simulink library "hapsrav_library"  (R2017a)
settings: Solver=VariableStepAuto  StartTime=0.0  StopTime=10.0  RelTol=1e-3
values from neighbouring files (symbols this model uses):
  absorb_h = 0:100:40000    [EnergySim.m]
  Adisk = pi * v.R_prop^2    [EnergySim.m]
  alpha_h = absorb_h    [EnergySim.m]
  aoa_data = zeros(n_cl, n)    [EnergySim.m]
  cl_bp = linspace(min_cl, max_cl,n_cl)    [EnergySim.m]
  D = [1       -.0065      288.15          0                   101325 ... (first row only)    [EnergySim.m]    (also in msn_params.m = sqrt((from_x - to_x)^2 + (from_y - to_y)^2); solar_vector.m = time.day + ut_time)
  d2r = pi / 180    (= 0.0174532925199)    [EnergySim.m]    (also in example1.m; example2.m; example3.m; example4.m)
  d_init = sqrt(dx*dx + dy*dy)    [EnergySim.m]    (also in msn_init.m)
  dchi0 = atan2(sin(dchi0), cos(dchi0))    [EnergySim.m]    (also in msn_init.m)
  dT = 0.5    [EnergySim.m]
  dT_fixed = 0.5    [EnergySim.m]
  dT_trig = 30    [EnergySim.m]
  earth_rho = 6378137.0    (= 6378137)    [EnergySim.m]
  fp = solarFP(p.orbit_rho, p.min_axis, p.orbit_dir, ic.x_ctr, ic.y_ctr, sun_az_0)    [EnergySim.m]    (also in load_fp.m = gid_tc(msn_idx).fp; solarFP.m = [1	6	2	nul eul 0	0	0	0	1	0)
  fp_coords = [x_entry y_entry]    [msn_params.m]
  fp_courses = [chi_adj nxt_chi dchi]    [msn_params.m]
  g = 9.80665    [EnergySim.m]
  Gsolar = 1367    [EnergySim.m]
  k = k+1    (= 5)    [EnergySim.m]
  K = D(:,2)    [EnergySim.m]
  lat_init = ic.lat_init_deg * obj.d2r    [EnergySim.m]
  M = time.month    [solar_vector.m]
  max_cl = max(cl_data(:))    [EnergySim.m]
  min_cl = min(cl_data(:))    [EnergySim.m]
  ND2 = load(fullfile(pwd,'nd2_data.mat'))    [EnergySim.m]    (also in nd2_data.mat = [0.0999999999999 0.200000000001 0.3 0.4 0.499999999998 0.700)
  next_init = fp(init_wp, 3)    [EnergySim.m]    (also in msn_init.m)
  pE_init = ic.pE_init    [EnergySim.m]
  pN_init = ic.pN_init    [EnergySim.m]
  r2d = 180 / pi    (= 57.2957795131)    [EnergySim.m]    (also in example1.m; example2.m; example3.m; example4.m)
  rho_SL = 1.225    [EnergySim.m]
  S = 110.4    [EnergySim.m]
  thr_lo_lim = 0.0    (= 0)    [EnergySim.m]
  time_init = struct('year', time.year, 'month', time.month,                  'day', time.day, 'hour', time.hour, 'min', time.min,                  'UTC', time.UTC)    [EnergySim.m]
  to_init = fp(init_wp, 1)    [EnergySim.m]    (also in msn_init.m)
  vgnd_init = sqrt(Vg)    [EnergySim.m]
  vtas_init = veas_init * sqrt(rho_sl/rho_alt)    [EnergySim.m]
  w_alt = 2.0 * w_alt    [EnergySim.m]
  w_xtrack = 2.0 * w_xtrack    [EnergySim.m]
undefined symbols (not defined in the file or in its folder): alpha, alpha_bp, alpha_circ, alt0_rate_init, alt_bp, alt_cmd_mode, alt_init, alt_lim_h, alt_lim_l, alt_rt_lim_periodic, cd_data, charge_eff, chi0_rate_init, chi_cmd_mode, chi_inf, chi_init, cl_data, discharge_eff, DiscIntNeverNeededParam, E_batt_max, E_init, Earth, enableFuzzyLogic, entry_init, epsln, epsln_circ, exit_init, f8_azimuth_offset, fig_eight_time, fp0, fp_coords0, fp_courses0, gamma_lim, hold_time, k_c, K_circ, lat_init_deg, lon_init_deg, max_alpha_bp, max_alt_bp, min_alpha_bp, min_alt_bp, min_axis, motor_eff, mppt_eff, num_motors, orb_dir_init, orb_len_init, orbit_dir, orbit_rho, P_acc, panel_eff, panel_vecs, phi_0, phi_lim, phi_lim_alt, phi_lim_alt_max, phi_lim_alt_min, phi_rt_lim, prop_eff_scale ... (+39)
libraries: simulink x59, hapsrav_library x9, fuzblock x3, atmospheric_library x1, aerolibtransform2 x1
(part 5 of 6)

== system hapsrav_library/hapsrav_main/Kinematic 6DOF/Selectable Modes/Waypoint_Navigation/Altitude/alt_rate ==
  max_clmb_rt : Inport
  max_desc_rt : Inport  Port=2
  d2alt : Inport  Port=3
  altRt0 : Inport  Port=4
  idleDesc : Inport  Port=5
  Constant : Constant  Value=dT
  Freezable Limited Integration1 : hapsrav_library/Freezable Limited Integration
  Mux : Mux  Inputs=2
  Scope : Scope
  d1alt : Outport
  wires:
  [dn_lim] -> Freezable Limited Integration1/6
  max_clmb_rt/1 -> [up_lim]
  max_desc_rt/1 -> [dn_lim]
  idleDesc/1 -> Freezable Limited Integration1/4
  altRt0/1 -> Freezable Limited Integration1/3
  [up_lim] -> Freezable Limited Integration1/5
  Constant/1 -> Freezable Limited Integration1/2
  d2alt/1 -> Freezable Limited Integration1/1
  Freezable Limited Integration1/1 -> Mux/1, d1alt/1
  Mux/1 -> Scope/1
  [dn_lim] -> Mux/2

== system hapsrav_library/hapsrav_main/Kinematic 6DOF/Selectable Modes/Waypoint_Navigation/Course/Circular Integration ==
  u : Inport
  x0 : Inport  Port=2
  Discrete-Time Integrator : DiscreteIntegrator  Commented=on  IntegratorMethod=Integration: Trapezoidal  InitialConditionSource=external  InitialConditionSetting=State (most efficient)  SampleTime=-1  ICPrevOutput=DiscIntNeverNeededParam  ICPrevScaledInput=DiscIntNeverNeededParam
  Integrator : Integrator  InitialConditionSource=external  WrapState=on
  Trigonometric Function : Trigonometry  Commented=on  Operator=sincos
  Trigonometric Function1 : Trigonometry  Commented=on  Operator=atan2
  y : Outport
  wires:
  Integrator/1 -> y/1
  u/1 -> Integrator/1
  x0/1 -> Integrator/2
  Discrete-Time Integrator/1 -> Trigonometric Function/1
  Trigonometric Function/2 -> Trigonometric Function1/2
  Trigonometric Function/1 -> Trigonometric Function1/1

== system hapsrav_library/hapsrav_main/Kinematic 6DOF/Selectable Modes/Waypoint_Navigation/Course/Rate Limits ==
  Vg : Inport
  alt : Inport  Port=2
  d2chi : Inport  Port=3
  d1Vg : Inport  Port=4
  Divide : Product  Inputs=*/
  Divide1 : Product  Inputs=*/
  Divide2 : Product  Inputs=**
  Divide3 : Product  Inputs=**
  Gain : Gain  Gain=g
  Gain1 : Gain  Gain=g
  Gain2 : Gain  Gain=-1
  Math Function : Math  Operator=reciprocal  SaturateOnIntegerOverflow=on
  Math Function1 : Math  Operator=square  SaturateOnIntegerOverflow=on
  Math Function2 : Math  Operator=square  SaturateOnIntegerOverflow=on
  Saturation : Saturate  UpperLimit=phi_lim_alt_max  LowerLimit=phi_lim_alt_min
  Saturation Dynamic : simulink/Discontinuities/Saturation Dynamic  OutMin=[]  OutMax=[]  OutDataTypeStr=Inherit: Same as second input  OutDataType=fixdt(1, 16)  OutScaling=2^-10  DoSatur=off
  Sum : Sum  Inputs=|-+
  Trigonometric Function : Trigonometry  Operator=tan
  Trigonometric Function1 : Trigonometry  Operator=cos
  phi_lim LUT : Lookup_n-D  NumberOfTableDimensions=1  BreakpointsForDimension1=phi_lim_alt  Table=phi_lim  ExtrapMethod=Clip  DiagnosticForOutOfRangeInput=Error  RemoveProtectionInput=on  UseLastTableValue=on  InternalRulePriority=Speed  RndMeth=Simplest  InputSameDT=on
  phi_rt_lim LUT : Lookup_n-D  NumberOfTableDimensions=1  BreakpointsForDimension1=phi_lim_alt  Table=phi_rt_lim  ExtrapMethod=Clip  DiagnosticForOutOfRangeInput=Error  RemoveProtectionInput=on  UseLastTableValue=on  InternalRulePriority=Speed  RndMeth=Simplest  InputSameDT=on
  phi_lim : Outport
  d2chi_lim : Outport  Port=2
  wires:
  d2chi/1 -> Saturation Dynamic/2
  Saturation Dynamic/1 -> d2chi_lim/1
  [phi_lim] -> Trigonometric Function/1
  Trigonometric Function/1 -> Gain/1
  Gain/1 -> Divide/1
  Math Function2/1 -> Divide/2
  Vg/1 -> [Vg]
  [Vg] -> Math Function2/1
  Trigonometric Function1/1 -> Math Function/1
  Math Function/1 -> Math Function1/1
  Math Function1/1 -> Gain1/1
  Gain1/1 -> Divide1/1
  [Vg] -> Divide1/2
  Divide1/1 -> Divide2/2
  Divide2/1 -> Sum/2
  Sum/1 -> [up_lim]
  [up_lim] -> Saturation Dynamic/1
  [up_lim] -> Gain2/1
  Gain2/1 -> Saturation Dynamic/3
  Divide/1 -> Divide3/2
  Divide3/1 -> Sum/1
  alt/1 -> Saturation/1
  [alt] -> phi_lim LUT/1
  phi_lim LUT/1 -> [phi_lim]
  [phi_lim] -> Trigonometric Function1/1
  [alt] -> phi_rt_lim LUT/1
  phi_rt_lim LUT/1 -> [phi_rt_lim]
  [phi_rt_lim] -> Divide2/1
  [phi_lim] -> phi_lim/1
  Saturation/1 -> [alt]
  d1Vg/1 -> Divide3/1

== system hapsrav_library/hapsrav_main/Kinematic 6DOF/Selectable Modes/Waypoint_Navigation/Course/Wrap +//- pi ==
  ang : Inport
  Trigonometric Function : Trigonometry  Operator=sincos
  Trigonometric Function1 : Trigonometry  Operator=atan2
  ang_pi : Outport
  wires:
  ang/1 -> Trigonometric Function/1
  Trigonometric Function/1 -> Trigonometric Function1/1
  Trigonometric Function/2 -> Trigonometric Function1/2
  Trigonometric Function1/1 -> ang_pi/1

== system hapsrav_library/hapsrav_main/Kinematic 6DOF/Selectable Modes/Waypoint_Navigation/Course/chi_dot ==
  Vg : Inport
  phi_lim : Inport  Port=2
  d2chi : Inport  Port=3
  Constant : Constant  Value=dT
  Constant1 : Constant  Value=g
  Constant2 : Constant  Value=chi0_rate_init
  Delay1 : Delay  DelayLength=1  InitialConditionSource=Input port
      settings: InputPortMap=u0,p4
  Divide : Product  Inputs=*/
  Divide1 : Product  Inputs=**
  Divide2 : Product  Inputs=**
  Gain : Gain  Gain=1/g
  Limited Integration : MATLAB Function  TreatAsAtomicUnit=on
  Trigonometric Function : Trigonometry  Operator=tan
  Trigonometric Function1 : Trigonometry  Operator=atan
  phi : Outport
  d1chi : Outport  Port=2
  wires:
  Constant/1 -> Limited Integration/2(T)
  Delay1/1 -> Limited Integration/4(x0)
  Limited Integration/2(x1) -> Delay1/1
  Limited Integration/1(y0) -> d1chi/1, Divide2/1
  d2chi/1 -> Limited Integration/1(u)
  Constant1/1 -> Divide/1
  Divide/1 -> Divide1/1
  phi_lim/1 -> Trigonometric Function/1
  Trigonometric Function/1 -> Divide1/2
  Divide1/1 -> [rate_lim]
  [rate_lim] -> Limited Integration/3(lim)
  Vg/1 -> [Vg]
  [Vg] -> Divide/2
  [Vg] -> Divide2/2
  Divide2/1 -> Gain/1
  Gain/1 -> Trigonometric Function1/1
  Trigonometric Function1/1 -> phi/1
  Constant2/1 -> Delay1/2

== system hapsrav_library/hapsrav_main/Kinematic 6DOF/Selectable Modes/Waypoint_Navigation/Lat Cmd Filter/Filtered Command ==
  chi cmd : Inport
  chi_init : Inport  Port=2
  Enable : EnablePort
  1/tau : Gain  Gain=0.1
  Delay1 : Delay  DelayLength=1  InitialConditionSource=Input port
      settings: InputPortMap=u0,p4
  Discrete-Time Integrator : DiscreteIntegrator  IntegratorMethod=Integration: Trapezoidal  InitialConditionSource=external  InitialConditionSetting=State (most efficient)  SampleTime=-1  ICPrevOutput=DiscIntNeverNeededParam  ICPrevScaledInput=DiscIntNeverNeededParam
  Sum : Sum  Inputs=|+-
  filt chi cmd : Outport
  wires:
  chi cmd/1 -> Sum/1
  [chi_init] -> Delay1/2
  1/tau/1 -> Discrete-Time Integrator/1
  chi_init/1 -> [chi_init]
  Sum/1 -> 1/tau/1
  Discrete-Time Integrator/1 -> filt chi cmd/1, Delay1/1
  [chi_init] -> Discrete-Time Integrator/2
  Delay1/1 -> Sum/2

== system hapsrav_library/hapsrav_main/Kinematic 6DOF/Selectable Modes/Waypoint_Navigation/Lat Cmd Filter/Unfiltered Command ==
  cmd : Inport
  Enable : EnablePort
  cmdFilt : Outport
  wires:
  cmd/1 -> cmdFilt/1

== system hapsrav_library/Cmd - Parametric/Chi Cmd/Flight Plan/Mission Command/Entry Mode/Desired Course/Desired Course ==
  xtrack : Inport
  Gain3 : Gain  Gain=k
  Gain5 : Gain  Gain=2/pi
  Gain6 : Gain  Gain=chi_inf
  Gain7 : Gain  Gain=-1
  Trigonometric Function1 : Trigonometry  Operator=atan
  chi_d : Outport
  wires:
  Gain7/1 -> chi_d/1
  Gain6/1 -> Gain7/1
  Trigonometric Function1/1 -> Gain5/1
  Gain3/1 -> Trigonometric Function1/1
  Gain5/1 -> Gain6/1
  xtrack/1 -> Gain3/1

== system hapsrav_library/Cmd - Parametric/Chi Cmd/Flight Plan/Mission Command/Entry Mode/xtrack Error/Distance ==
  to_x : Inport
  from_x : Inport  Port=2
  to_y : Inport  Port=3
  from_y : Inport  Port=4
  Product of Elements : Product
  Product of Elements1 : Product
  Sqrt : Sqrt  SaturateOnIntegerOverflow=on
  Sum : Sum  Inputs=|+-
  Sum1 : Sum  Inputs=|+-
  Sum2 : Sum  Inputs=|++
  Dist : Outport
  wires:
  Sum1/1 -> [dy]
  to_x/1 -> Sum/1
  Sum/1 -> [dx]
  from_y/1 -> Sum1/2
  to_y/1 -> Sum1/1
  Sqrt/1 -> Dist/1
  Sum2/1 -> Sqrt/1
  [dx] -> Product of Elements/1, Product of Elements/2
  Product of Elements1/1 -> Sum2/2
  Product of Elements/1 -> Sum2/1
  [dy] -> Product of Elements1/1, Product of Elements1/2
  from_x/1 -> Sum/2

== system hapsrav_library/Cmd - Parametric/Chi Cmd/Flight Plan/Mission Command/Not Entry Mode/Circular Pattern Holding/Sweep Angle ==
  av_y : Inport
  y_ctr : Inport  Port=2
  av_x : Inport  Port=3
  x_ctr : Inport  Port=4
  Abs : Abs
  Abs1 : Abs
  Abs2 : Abs
  Counter Free-Running : simulink/Sources/Counter Free-Running  NumBits=32  tsamp=-1
  Delay : Delay  DelayLength=1  InitialConditionSource=Input port
      settings: InputPortMap=u0,p4
  Memory : Memory
  Memory3 : Memory
  Sum1 : Sum  Inputs=|+-
  Sum2 : Sum  Inputs=|+-
  Sum3 : Sum  Inputs=|+-
  Sum4 : Sum  Inputs=|++
  Switch : Switch  Criteria=u2 ~= 0
  Trigonometric Function1 : Trigonometry  Operator=atan2
  swept_angle : Outport
  wires:
  Memory/1 -> Sum4/2
  Abs/1 -> Delay/2
  Sum1/1 -> Abs2/1
  [rel_hdg] -> Switch/3
  Sum3/1 -> Trigonometric Function1/1
  Abs2/1 -> Sum4/1
  Trigonometric Function1/1 -> [rel_hdg]
  Sum2/1 -> Trigonometric Function1/2
  [rel_hdg] -> Abs1/1
  Sum4/1 -> Memory/1, swept_angle/1
  Delay/1 -> Sum1/2
  [rel_hdg_0] -> Abs/1
  Counter Free-Running/1 -> Switch/2
  y_ctr/1 -> Sum3/2
  av_x/1 -> Sum2/1
  x_ctr/1 -> Sum2/2
  av_y/1 -> Sum3/1
  Abs1/1 -> Sum1/1, Delay/1
  Memory3/1 -> Switch/1
  Switch/1 -> Memory3/1, [rel_hdg_0]

== system hapsrav_library/Cmd - Parametric/Chi Cmd/Flight Plan/Mission Command/Not Entry Mode/Linear Following/Path Following ==
  leg_coords : Inport
  leg_crs : Inport  Port=2
  av_state : Inport  Port=3
  Bus Selector1 : BusSelector  OutputSignals=av_posn,av_course,av_gndspeed
  Constant1 : Constant  Value=alpha
  Constant2 : Constant  Value=epsln
  Constant3 : Constant  Value=k
  Constant4 : Constant  Value=K
  Constant5 : Constant  Value=chi_inf
  Course : Subsystem  TreatAsAtomicUnit=on
  Desired Course : Subsystem  TreatAsAtomicUnit=on
  Logical Operator : Logic  Operator=NOT  AllPortsSameDT=off  OutDataTypeStr=boolean
  MATLAB Function : MATLAB Function  TreatAsAtomicUnit=on
  Merge1 : Merge
  xtrack Error : Subsystem  TreatAsAtomicUnit=on
  chi_cmd : Outport
  chi_d : Outport  Port=2
  xtrack : Outport  Port=3
  wires:
  [chi_d] -> chi_d/1
  Merge1/1 -> [chi_d]
  [chi_d_0] -> Merge1/2
  [chi_d_1] -> Merge1/1
  Course/1(chi_d) -> [chi_d_0]
  [av_posn] -> Course/2(av_posn)
  [leg_coords] -> Course/1(leg_coords)
  [leg_coords] -> xtrack Error/1(leg_coords)
  leg_coords/1 -> [leg_coords]
  [collocated] -> Course/Enable
  [collocated] -> Logical Operator/1
  Logical Operator/1 -> Desired Course/Enable
  xtrack Error/2(collacated) -> [collocated]
  leg_crs/1 -> Desired Course/1(leg_crs)
  [xtrack] -> xtrack/1
  [xtrack] -> Desired Course/2(xtrack)
  Desired Course/1(chi_d) -> [chi_d_1]
  xtrack Error/1(xtrk) -> [xtrack]
  [av_posn] -> xtrack Error/2(av_posn)
  Bus Selector1/1 -> [av_posn]  "<av_posn>"
  [Vg] -> MATLAB Function/4(Vg)
  [chi] -> MATLAB Function/1(chi)
  Bus Selector1/3 -> [Vg]  "<av_gndspeed>"
  av_state/1 -> Bus Selector1/1
  Bus Selector1/2 -> [chi]  "<av_course>"
  Constant5/1 -> MATLAB Function/5(chi_inf)
  Constant3/1 -> MATLAB Function/8(k)
  [chi_d] -> MATLAB Function/2(chi_d)
  [xtrack] -> MATLAB Function/3(xtrack)
  Constant2/1 -> MATLAB Function/7(e)
  Constant1/1 -> MATLAB Function/6(alpha)
  Constant4/1 -> MATLAB Function/9(K)
  MATLAB Function/1(chi_cmd) -> chi_cmd/1

== system hapsrav_library/Cmd - Parametric/Chi Cmd/Flight Plan/Mission Director/Nav Leg/Flight Plan/Realtime FP ==
  sol_az : Inport  PortDimensions=1
  Enable : EnablePort
  Constant4 : Constant  Value=orbit_rho  VectorParams1D=off  OutDataTypeStr=double
  Constant5 : Constant  Value=min_axis  VectorParams1D=off  OutDataTypeStr=double
  Constant6 : Constant  Value=orbit_dir  VectorParams1D=off  OutDataTypeStr=boolean
  Constant7 : Constant  Value=x_ctr  VectorParams1D=off  OutDataTypeStr=double
  Constant8 : Constant  Value=y_ctr  VectorParams1D=off  OutDataTypeStr=double
  MATLAB Function : MATLAB Function  TreatAsAtomicUnit=on
  Trigonometric Function : Trigonometry  Operator=sincos  OutputSignalType=real
  Trigonometric Function1 : Trigonometry  Operator=atan2  OutputSignalType=real
  fp : Outport  PortDimensions=[6,11]  InitialOutput=fp0
  fp_courses : Outport  Port=2  PortDimensions=[6,3]  InitialOutput=fp_courses0
  fp_coords : Outport  Port=3  PortDimensions=[6,2]  InitialOutput=fp_coords0
  wires:
  sol_az/1 -> Trigonometric Function/1
  MATLAB Function/3(fp_coords) -> fp_coords/1
  MATLAB Function/2(fp_courses) -> fp_courses/1
  Trigonometric Function1/1 -> MATLAB Function/6(az)
  Trigonometric Function/2 -> Trigonometric Function1/2
  Trigonometric Function/1 -> Trigonometric Function1/1
  Constant8/1 -> MATLAB Function/5(y_ctr)
  Constant5/1 -> MATLAB Function/2(min_axis)
  Constant7/1 -> MATLAB Function/4(x_ctr)
  Constant4/1 -> MATLAB Function/1(maj_axis)
  Constant6/1 -> MATLAB Function/3(orbit_dir)
  MATLAB Function/1(fp) -> fp/1

== system hapsrav_library/Cmd - Parametric/Chi Cmd/Flight Plan/Mission Director/Nav Leg/WP Coords/Course ==
  to wp : Inport
  fp_courses : Inport  Port=2
  Assignment1 : Assignment  DiagnosticForDimensions=Warning  IndexOptions=Index vector (port)  Indices=1  OutputSizes=1
  Constant3 : Constant  Value=sel_vec
  Constant4 : Constant
  Demux1 : Demux  Outputs=3
  Gain1 : Gain  Commented=on  Gain=fp_courses  Multiplication=Matrix(u*K)
  Product : Product  Multiplication=Matrix(*)
  Reshape : Reshape  OutputDimensionality=Row vector (2-D)
  Terminator : Terminator
  Terminator1 : Terminator
  next_leg_crs : Outport
  wires:
  fp_courses/1 -> Product/2
  Product/1 -> Demux1/1
  Reshape/1 -> Product/1
  Assignment1/1 -> Reshape/1
  Demux1/3 -> Terminator1/1  "delta_crs"
  to wp/1 -> Assignment1/3
  Constant3/1 -> Assignment1/1
  Constant4/1 -> Assignment1/2
  Demux1/2 -> next_leg_crs/1
  Demux1/1 -> Terminator/1  "leg_crs"

== system hapsrav_library/Cmd - Parametric/Chi Cmd/Flight Plan/Mission Director/Nav Leg/WP Coords/From WP ==
  to wp : Inport
  fp_coords : Inport  Port=2
  Assignment1 : Assignment  DiagnosticForDimensions=Warning  IndexOptions=Index vector (port)  Indices=1  OutputSizes=1
  Constant3 : Constant  Value=sel_vec
  Constant4 : Constant
  Demux1 : Demux  Outputs=2
  Gain1 : Gain  Commented=on  Gain=fp_coords  Multiplication=Matrix(u*K)
  Product : Product  Multiplication=Matrix(*)
  Reshape : Reshape  OutputDimensionality=Row vector (2-D)
  out_x : Outport
  out_y : Outport  Port=2
  wires:
  fp_coords/1 -> Product/2
  Product/1 -> Demux1/1
  Reshape/1 -> Product/1
  Assignment1/1 -> Reshape/1
  to wp/1 -> Assignment1/3
  Constant3/1 -> Assignment1/1
  Constant4/1 -> Assignment1/2
  Demux1/2 -> out_y/1
  Demux1/1 -> out_x/1

== system hapsrav_library/Cmd - Parametric/Chi Cmd/Flight Plan/Mission Director/Nav Leg/WP Coords/To WP ==
  to wp : Inport
  fp_coords : Inport  Port=2
  Assignment1 : Assignment  DiagnosticForDimensions=Warning  IndexOptions=Index vector (port)  Indices=1  OutputSizes=1
  Constant3 : Constant  Value=sel_vec
  Constant4 : Constant
  Demux1 : Demux  Outputs=2
  Gain1 : Gain  Commented=on  Gain=fp_coords  Multiplication=Matrix(u*K)
  Product : Product  Multiplication=Matrix(*)
  Reshape : Reshape  OutputDimensionality=Row vector (2-D)
  out_x : Outport
  out_y : Outport  Port=2
  wires:
  Product/1 -> Demux1/1
  fp_coords/1 -> Product/2
  Reshape/1 -> Product/1
  Assignment1/1 -> Reshape/1
  Demux1/1 -> out_x/1
  Demux1/2 -> out_y/1
  Constant4/1 -> Assignment1/2
  Constant3/1 -> Assignment1/1
  to wp/1 -> Assignment1/3

== system hapsrav_library/Cmd - Parametric/Chi Cmd/Flight Plan/Mission Command/Not Entry Mode/Linear Following/Path Following/Course ==
  leg_coords : Inport
  av_posn : Inport  Port=2
  Enable : EnablePort
  Demux1 : Demux
  Demux2 : Demux
  Sum : Sum  Inputs=|+-
  Sum1 : Sum  Inputs=|+-
  Terminator{,1..3} (4 alike) : Terminator
  Trigonometric Function : Trigonometry  Operator=atan2
  chi_d : Outport
  wires:
  Trigonometric Function/1 -> chi_d/1
  Sum1/1 -> Trigonometric Function/2
  Sum/1 -> Trigonometric Function/1
  [av_x] -> Sum1/2
  [x1] -> Sum1/1
  [av_y] -> Sum/2
  [y1] -> Sum/1
  Demux1/4 -> Terminator1/1
  Demux1/3 -> Terminator/1
  av_posn/1 -> Demux1/1
  Demux1/2 -> [av_y]
  Demux1/1 -> [av_x]
  leg_coords/1 -> Demux2/1
  Demux2/4 -> Terminator3/1
  Demux2/3 -> Terminator2/1
  Demux2/2 -> [y1]
  Demux2/1 -> [x1]

== system hapsrav_library/Cmd - Parametric/Chi Cmd/Flight Plan/Mission Command/Not Entry Mode/Linear Following/Path Following/Desired Course ==
  leg_crs : Inport
  xtrack : Inport  Port=2
  Enable : EnablePort
  Desired Course : Subsystem
  Sum : Sum  Inputs=|++
  chi_d : Outport
  wires:
  leg_crs/1 -> Sum/1
  xtrack/1 -> Desired Course/1(xtrack)
  Sum/1 -> chi_d/1
  Desired Course/1(chi_d) -> Sum/2

== system hapsrav_library/Cmd - Parametric/Chi Cmd/Flight Plan/Mission Command/Not Entry Mode/Linear Following/Path Following/xtrack Error ==
  leg_coords : Inport
  av_posn : Inport  Port=2
  Compare To Constant : simulink/Logic and Bit Operations/Compare To Constant  relop=<=  const=10  OutDataTypeStr=boolean
  Demux1 : Demux
  Demux2 : Demux
  Distance : Subsystem  TreatAsAtomicUnit=on
  MATLAB Function : MATLAB Function  TreatAsAtomicUnit=on
  Product{,1..3} (4 alike) : Product
  Sum{,1..2,4} (4 alike) : Sum  Inputs=|+-
  Sum3 : Sum  Inputs=|++
  Terminator : Terminator
  Terminator1 : Terminator
  xtrk : Outport
  collacated : Outport  Port=2
  wires:
  Compare To Constant/1 -> collacated/1
  leg_coords/1 -> Demux2/1
  Demux1/4 -> Terminator1/1
  Demux1/3 -> Terminator/1
  Demux2/4 -> [y2]
  Demux2/3 -> [x2]
  Demux2/2 -> [y1]
  Demux2/1 -> [x1]
  av_posn/1 -> Demux1/1
  Demux1/2 -> [av_y]
  Demux1/1 -> [av_x]
  Distance/1(Dist) -> MATLAB Function/2(den), Compare To Constant/1
  [y2] -> Distance/4(from_y)
  [y1] -> Distance/3(to_y)
  [x2] -> Distance/2(from_x)
  [x1] -> Distance/1(to_x)
  MATLAB Function/1(xtrack) -> xtrk/1
  Sum4/1 -> MATLAB Function/1(num)
  Sum2/1 -> Sum3/1
  Product2/1 -> Sum3/2
  Product/1 -> Sum2/1
  [av_x] -> Product/2
  [y2] -> Sum1/1
  [av_y] -> Product1/2
  [x1] -> Sum/2
  [x1] -> Product3/2
  [y2] -> Product3/1
  [x2] -> Sum/1
  [dx] -> Product1/1
  [dy] -> Product/1
  Sum3/1 -> Sum4/1
  [x2] -> Product2/1
  Product1/1 -> Sum2/2
  Sum1/1 -> [dy]
  [y1] -> Sum1/2
  Sum/1 -> [dx]
  Product3/1 -> Sum4/2
  [y1] -> Product2/2

== system hapsrav_library/Cmd - Parametric/Chi Cmd/Flight Plan/Mission Command/Not Entry Mode/Linear Following/Path Following/Desired Course/Desired Course ==
  xtrack : Inport
  Gain3 : Gain  Gain=k
  Gain5 : Gain  Gain=2/pi
  Gain6 : Gain  Gain=chi_inf
  Gain7 : Gain  Gain=-1
  Trigonometric Function1 : Trigonometry  Operator=atan
  chi_d : Outport
  wires:
  Gain7/1 -> chi_d/1
  Gain6/1 -> Gain7/1
  Trigonometric Function1/1 -> Gain5/1
  Gain3/1 -> Trigonometric Function1/1
  Gain5/1 -> Gain6/1
  xtrack/1 -> Gain3/1

== system hapsrav_library/Cmd - Parametric/Chi Cmd/Flight Plan/Mission Command/Not Entry Mode/Linear Following/Path Following/xtrack Error/Distance ==
  to_x : Inport
  from_x : Inport  Port=2
  to_y : Inport  Port=3
  from_y : Inport  Port=4
  Product of Elements : Product
  Product of Elements1 : Product
  Sqrt : Sqrt  SaturateOnIntegerOverflow=on
  Sum : Sum  Inputs=|+-
  Sum1 : Sum  Inputs=|+-
  Sum2 : Sum  Inputs=|++
  Dist : Outport
  wires:
  Sum1/1 -> [dy]
  to_x/1 -> Sum/1
  Sum/1 -> [dx]
  from_y/1 -> Sum1/2
  to_y/1 -> Sum1/1
  Sqrt/1 -> Dist/1
  Sum2/1 -> Sqrt/1
  [dx] -> Product of Elements/1, Product of Elements/2
  Product of Elements1/1 -> Sum2/2
  Product of Elements/1 -> Sum2/1
  [dy] -> Product of Elements1/1, Product of Elements1/2
  from_x/1 -> Sum/2

== matlab function hapsrav_library/Cmd - Parametric/Chi Cmd/Flight Plan/Mission Command/Not Entry Mode/Circular Pattern Holding/MATLAB Function1 ==
  data: av_x input; av_y input; d output; x_c input; y_c input; orbit_dir input; g output; beta output; r_c input; chi_d output; k_c input
function [d,g,beta,chi_d] = relPosn(av_x, av_y, x_c, y_c, orbit_dir, r_c, k_c)

x = av_x;
y = av_y;
% x_c = to_x
% y_c = to_y;

dx = x - x_c;
dy = y - y_c;

d = sqrt(dx * dx + dy * dy);
g = atan2(dy, dx);       % correct as dy, dx

ang_y = k_c * (d - r_c);
ang_x = r_c;

if (orbit_dir)
    % CCW
    chi_d = g - pi/2 - atan(ang_y/ ang_x);
else
    % CW
    chi_d = g + pi/2 + atan(ang_y/ ang_x);
end

chi_d = wrap2pi(chi_d);

% Compute beta
d_err = d - r_c;
k_r = k_c / r_c;
beta = k_r / (1 + (k_r * d_err)^2);


end

function wrpd = wrap2pi(angl)

% Wrap to +/- pi
if (angl > pi)
    wrpd = -pi + (angl - pi);
elseif (angl < -pi)
    wrpd = 2 * pi + angl;
else
    wrpd = angl;
end

end

== matlab function hapsrav_library/Freezable Limited Integration/Limited Integration ==
  data: u input; y0 output; T input; uplim input; lolim input; x0 input; x1 output
function [y0,x1] = lim_integr(u, T, uplim, lolim, x0)

K = 1.0;

y0   = x0 + K * T/2 * u;
y0 = max(min(y0, uplim), lolim);
x1   = y0 + K * T/2 * u;

end

== stateflow chart hapsrav_library/hapsrav_main/Kinematic 6DOF/Idle Pwr/Decel Detection ==
  state Steady
    entry:
    spd_flag = 0
    idleDecel = 0
  state Decel
    entry: spd_flag = -1
    state powered_decel
      entry: idleDecel = 0
    state idle_decel
      entry: idleDecel = 1
    (default) -> powered_decel
    powered_decel -> idle_decel : [thrust < 10]
  state Accel
    entry:
    spd_flag = 1
    idleDecel = 0
  (default) -> Steady
  Steady -> Accel [order 1] : [vdot > 0.01]
  Steady -> Decel [order 2] : [vdot < -0.01]
  Decel -> Steady : [vdot > 0.0]
  Accel -> Steady : [vdot <= 0.01]
  data: vdot input; thrust input; spd_flag output; idleDecel output

== stateflow chart hapsrav_library/hapsrav_main/Kinematic 6DOF/Idle Pwr/Descent Detection ==
  state Level
    entry:
    alt_flag = 0
    idleDesc = 0
  state Descending
    entry: alt_flag = -1
    state powered_descent
      entry: idleDesc = 0
    state idle_descent
      entry: idleDesc = 1
    (default) -> powered_descent
    idle_descent -> powered_descent : [thrust>13]
    powered_descent -> idle_descent : [thrust<10]
  state Climbing
    entry:
    alt_flag = 1
    idleDesc = 0
  (default) -> Level
  Level -> Climbing [order 1] : [hdot > 0.05]
  Level -> Descending [order 2] : [hdot < -0.05]
  Descending -> Level : [hdot >= -0.05]
  Climbing -> Level : [hdot <= 0.05]
  data: hdot input; thrust input; alt_flag output; idleDesc output

== matlab function hapsrav_library/Cmd - Parametric/Chi Cmd/Flight Plan/Mission Command/Not Entry Mode/Circular Pattern Holding/MATLAB Function3 ==
  data: chi input; chi_cmd output; d input; g input; chi_d input; beta input; Vg input; alpha input; e input; K input
function chi_cmd = chiCmdCirc(chi, d, g, chi_d, beta, Vg, alpha, e, K)

chi_err = wrap2pi(chi - chi_d);
angl = chi - g;
angl = wrap2pi(angl);

chi_cmd = chi + Vg * sin(angl) / alpha / d;
chi_cmd = chi_cmd - beta * Vg * cos(angl) / alpha;

satVal = sat_val(chi_err, e);
chi_cmd = chi_cmd - K * satVal / alpha;
chi_cmd = wrap2pi(chi_cmd);

end

function satVal = sat_val(u,epsln)

x = u / epsln;

if (abs(x) <= 1)
    satVal = x;
else
    satVal = sign(x);
end

end

function wrpd = wrap2pi(angl)

% Wrap to +/- pi
if (angl > pi)
    wrpd = -pi + (angl - pi);
elseif (angl < -pi)
    wrpd = 2 * pi + angl;
else
    wrpd = angl;
end

end

== matlab function hapsrav_library/hapsrav_main/Kinematic 6DOF/Selectable Modes/Trajectory_Optimization/Vert Cmd Filter/Limited Integration ==
  data: u input; y0 output; T input; uplim input; lolim input; x0 input; x1 output
function [y0,x1] = lim_integr(u, T, uplim, lolim, x0)

K = 1.0;

y0   = x0 + K * T/2 * u;
y0 = max(min(y0, uplim), lolim);
x1   = y0 + K * T/2 * u;

end

== matlab function hapsrav_library/Cmd - Parametric/Chi Cmd/Flight Plan/Mission Command/Not Entry Mode/Linear Following/Path Following/MATLAB Function ==
  data: chi input; chi_cmd output; chi_d input; xtrack input; Vg input; chi_inf input; alpha input; e input; k input; K input
function chi_cmd = chi_cmd_fcn(chi, chi_d, xtrack, Vg, chi_inf, alpha, e, k, K)

chi_err = wrap2pi(chi - chi_d);

a = chi_inf * 2 / alpha / pi;
b = k / (1 + (k*xtrack)^2);

chi_cmd = chi - a * b * Vg * sin(chi);

satVal = sat_val(chi_err, e);

chi_cmd = chi_cmd - K * satVal / alpha;

% Command should probably be limited
chi_cmd = wrap2pi(chi_cmd);

end

function satVal = sat_val(u,epsln)

x = u / epsln;

if (abs(x) <= 1)
    satVal = x;
else
    satVal = sign(x);
end

end

function wrpd = wrap2pi(angl)

% Wrap to +/- pi
if (angl > pi)
    wrpd = -pi + (angl - pi);
elseif (angl < -pi)
    wrpd = 2 * pi + angl;
else
    wrpd = angl;
end

end

== matlab function hapsrav_library/Cmd - Parametric/Chi Cmd/Flight Plan/Mission Command/Not Entry Mode/Linear Following/Path Following/xtrack Error/MATLAB Function ==
  data: num input; xtrack output; den input
function xtrack = fcn(num, den)

if (abs(den) <  0.01)
    xtrack = 0.0;
else
    xtrack = num / den;
end

end

== matlab function hapsrav_library/Cmd - Parametric/Chi Cmd/Flight Plan/Mission Command/Entry Mode/xtrack Error/MATLAB Function ==
  data: num input; xtrack output; den input
function xtrack = fcn(num, den)

if (abs(den) <  0.01)
    xtrack = 0.0;
else
    xtrack = num / den;
end

end

== matlab function hapsrav_library/Cmd - Parametric/Chi Cmd/Flight Plan/Mission Command/Entry Mode/MATLAB Function ==
  data: chi input; chi_cmd output; chi_d input; xtrack input; Vg input; chi_inf input; alpha input; e input; k input; K input
function chi_cmd = chi_cmd_fcn(chi, chi_d, xtrack, Vg, chi_inf, alpha, e, k, K)

chi_err = wrap2pi(chi - chi_d);

a = chi_inf * 2 / alpha / pi;
b = k / (1 + (k*xtrack)^2);

chi_cmd = chi - a * b * Vg * sin(chi);

satVal = sat_val(chi_err, e);

chi_cmd = chi_cmd - K * satVal / alpha;

% Command should probably be limited
chi_cmd = wrap2pi(chi_cmd);

end

function satVal = sat_val(u,epsln)

x = u / epsln;

if (abs(x) <= 1)
    satVal = x;
else
    satVal = sign(x);
end

end

function wrpd = wrap2pi(angl)

% Wrap to +/- pi
if (angl > pi)
    wrpd = -pi + (angl - pi);
elseif (angl < -pi)
    wrpd = 2 * pi + angl;
else
    wrpd = angl;
end

end

== stateflow chart hapsrav_library/hapsrav_main/Kinematic 6DOF/Power Model/Battery and Potential Management/Stateflow Battery Management ==
  state charge
    entry: ChargeMode=1;
  state hold
    entry: ChargeMode=0;
  state discharge
    entry: ChargeMode=-1;
  charge -> hold [order 1] : [E_batt >= E_batt_max]
  hold -> charge [order 2] : [P_el_net > 0 & E_batt < E_batt_max]
  charge -> hold [order 2] : [P_el_net <= 0]
  (default) -> hold
  discharge -> hold [order 1] : [E_batt <= 0]
  hold -> discharge [order 1] : [P_el_net < 0 & E_batt > 0]
  discharge -> hold [order 2] : [P_el_net >= 0]
  data: P_el_net input; E_batt input; ChargeMode output; E_batt_max parameter

== stateflow chart hapsrav_library/hapsrav_main/Kinematic 6DOF/Power Model/Battery and Potential Management/Stateflow Potential Management ==
  state climb
    entry: ClimbMode=1;
  state hold
    entry: ClimbMode=0;
  state descend
    state powered_descent
      entry: ClimbMode=-1;
    state glide
      entry: ClimbMode=-2;
    (default) -> powered_descent
    powered_descent -> glide : [P_el_in < 0.001*P_acc]
    glide -> powered_descent : [P_el_in > 0.001*P_acc*1.1]
  climb -> descend [order 2] : [P_el_in < P_cruise]
  descend -> climb [order 2] : [P_el_in > P_cruise*1.1]
  climb -> hold [order 1] : [alt >= alt_lim_h | E_batt < E_batt_max]
  hold -> climb [order 1] : [P_el_in > P_cruise*1.1 & alt < alt_lim_h & E_batt >= E_batt_max]
  (default) -> hold
  hold -> descend [order 2] : [P_el_in < P_cruise & alt > alt_lim_l]
  descend -> hold [order 1] : [alt <= alt_lim_l]
  data: P_cruise input; alt input; alt_lim_h parameter; ClimbMode output; E_batt input; E_batt_max parameter; alt_lim_l parameter; P_el_in input; P_acc parameter

== matlab function hapsrav_library/hapsrav_main/Kinematic 6DOF/Power Model/Electric Power In/atmos_absorb_adj/atmospheric adjustment ==
  data: h input; rel_power output; zth input; earth_rho input; alpha_h input; absorb_h input
function rel_power = sunpower(h, zth, earth_rho, alpha_h, absorb_h)

    Z_MAX = 1430;       % maximum raytrace distance, km (never need a ray longer than 1430 km)
    z = Z_MAX:-0.2:0;                   % initialize z-distance vector, in km; stepsize 0.2 km
    H_MIN = 0;          % minimum grazing altitude, km (mountains and hot air distortion get in the way below this altitude)

    ray_I = zeros(length(z),1);
    rel_power = 1;

    ray_I(1) = 1;      % initialize intensity at maximum distance
    ray_h = sqrt(z.^2 + (earth_rho + h)^2 + 2*(earth_rho + h) * z * cosd (zth) ) - earth_rho;  % calculate ray altitudes, in km
    dII=zeros(size(ray_h)); % initialize absorbances
    dII(1)=0;           % dII represents "dI/I", the transmission ratio at a given height

    dz=dII;             % differential distance in the ray direction z, in km
    dz(1)=0;            % set initial differential distance to zero

    for i=2:length(z)        % absorb the ray from Z_MAX (max distance) to 0 (aircraft)
        dz(i)=z(i-1)-z(i);   % differential distance in m

        if ray_h(i)>40
            dII(i) = 0;                 % assume no absorption above 40 km because the air is so thin
            ray_I(i) = ray_I(i-1);
        elseif ray_h(i)<H_MIN           % below a critical height, sun sets, no more tracing needed
            ray_I(i) = 0;               % force intensity to zero
            break;
        else
            dII(i) = interp1(absorb_h,alpha_h,ray_h(i)*1000); % interpolate dII in ratio per m
            ray_I(i) = ray_I(i-1) * exp( dII(i)*1000 * dz(i) );   
        end

    end
    
    if abs(zth) < 90
        rel_power = max([ray_I(i), 0]);
    else
        rel_power = 0;
    end
end

== matlab function hapsrav_library/hapsrav_main/Kinematic 6DOF/Power Model/Electric Power In/projected area/Projected area ==
  data: y input; p input; r input; proj_area output; panel_vecs input; sun_vector input
function proj_area = f(y, p, r, panel_vecs, sun_vector)
% given magnitudes and directions of solar panels in body coordinates
% (direction as unit vector [+fore; +right; +down]), transform to ned
% coordinates to find angle with solar vector
%
% multiply each panel's direction in ned by its area
sun_vector = reshape(sun_vector, [1,3]);

% body frame to ned frame (R_{b}^{v})
ypr = [cosd(y)*cosd(p) cosd(y)*sind(p)*sind(r)-cosd(r)*sind(y) sind(r)*sind(y)+cosd(y)*sind(p)*cosd(r);
       cosd(p)*sind(y) cosd(y)*cosd(r)+sind(y)*sind(p)*sind(r) sind(y)*sind(p)*cosd(r)-cosd(y)*sind(r);
       -sind(p)        cosd(p)*sind(r)                         cosd(p)*cosd(r)];

panels_ned = zeros(size(panel_vecs));
for i=1:length(panel_vecs)
    panels_ned(:,i) = ypr * panel_vecs(:,i);
end

dot_products = sun_vector * panels_ned;
dot_products_clipped = max(0, dot_products);

proj_area = sum(dot_products_clipped);
